simulink model "Longitudinal"  (R2025b)
settings: Solver=VariableStepAuto  StartTime=0.0  StopTime=5  MaxStep=0.001  RelTol=1e-3
undefined symbols (not defined in the file): car, rad, s, Tau_1, Tau_2, Tau_3, Tau_4, Tau_EM, tyre
libraries: aerolibconvert2 x3, simulink x2, autolibcoupling x1
(part 3 of 3)

== matlab function Longitudinal/longitudinal dynamics/Kinematics/Subsystem/Damper front/MATLAB Function ==
  data: x_dot input; x_dot_comp output; x_dot_reb output
function [ x_dot_comp , x_dot_reb ] = conv_x_dot(x_dot)

if x_dot > 0 
    x_dot_comp = x_dot; 
    x_dot_reb = 0;
else 
    x_dot_comp = 0;
    x_dot_reb = - x_dot;
end

== matlab function Longitudinal/longitudinal dynamics/Kinematics/Subsystem/Rear damping/MATLAB Function ==
  data: x_dot input; x_dot_comp output; x_dot_reb output
function [ x_dot_comp , x_dot_reb ] = conv_x_dot(x_dot)

if x_dot > 0 
    x_dot_comp = x_dot; 
    x_dot_reb = 0;
else 
    x_dot_comp = 0;
    x_dot_reb = - x_dot;
end

== matlab function Longitudinal/longitudinal dynamics/Fx equilibrium ==
  data: Drag output; Fz_FL output; a input; Fz_RR output; Fz_RL output; Fz_FR output; delta_Fz output; v input; Cx input; Cz input; delta_wb_front input; delta_wb_rear input; Jr_tot input; car input; M_inerzia output
function [Drag, Fz_FL, Fz_RR, Fz_RL, Fz_FR, delta_Fz, M_inerzia] = fx_equilibrium(a, v, Cx, Cz, delta_wb_front, delta_wb_rear, Jr_tot, car)

wb = car.wb0 + delta_wb_front + delta_wb_rear; %m

Downforce = 0.5 * car.rho * Cz * car.frontal_area * v ^ 2; % downforce N
Drag = 0.5 * car.rho * Cx * car.frontal_area * v ^ 2; % drag N
M_aero = Drag * (car.h_cp - car.h_cog) - Downforce * (car.lf - car.x_cp); %Nm

delta_Fz = Drag * car.h_cog / wb + M_aero / wb; %N
delta_Fz=delta_Fz/2;

M_inerzia = car.m * a * car.h_cog;
%J_f è di una singola ruota
%J_r totale da ruota a motore ICE
Fz_front = - Drag * car.h_cog / wb + (car.m * car.g + Downforce) * (car.lr + delta_wb_rear - car.delta) / wb - M_aero / wb - car.J_f*2* a / (car.R * wb); %N  (verificare J_f*4 oppure J_f*2!!!!!!!!!!!)

Fz_rear = Drag * car.h_cog / wb + (car.m * car.g + Downforce) * (car.lf + delta_wb_front + car.delta) / wb + M_aero / wb + Jr_tot * a / (car.R * wb); %N

if Fz_front <= 0
    Fz_rear = Fz_rear + Fz_front;
    Fz_front = 0;
elseif Fz_rear <0 
    Fz_front = Fz_front + Fz_rear;
    Fz_rear = 0;
end

Fz_FR = Fz_front / 2 ;
Fz_FL = Fz_FR ;

Fz_RL = Fz_rear / 2;
Fz_RR = Fz_RL ;

== matlab function Longitudinal/longitudinal dynamics/Fx powertrain calculation/FL ==
  data: Fx_EM_FL output; T input; T_b input; Fz input; a input; car input; delta_z_tyre_FL input
function Fx_EM_FL = fcn( T,T_b, Fz, a, car, delta_z_tyre_FL)

Fx_EM_FL = ( T - T_b - Fz * car.delta - car.J_f * a / ( car.R - delta_z_tyre_FL ) ) / ( car.R - delta_z_tyre_FL ) ; %N
% J - parameter for each tyre - J_f & J_r

== matlab function Longitudinal/Tyres/Rear Right ==
  data: tyre_RR input; Fx output; Fy output
function [Fx, Fy] = fcn(tyre_RR)

y = u;

== matlab function Longitudinal/Tyres/Front Right ==
  data: SR input; tyre input; Fx output; p input; Fz input; camber input
function Fx = fcn(SR,tyre,p,Fz,camber)

% PAC2002 puro longitudinale (Fx vs k)

     Fz0 = tyre.Fz0;
     if Fz0 == 0, Fz0 = max(1, Fz); end
    dfz = (Fz - Fz0)/Fz0;

    pi0 = tyre.pi0;  % Pa nominale
    dpi = (p - pi0)/pi0;
    
    Cx1 = tyre.Cx1;
    Dx1 = tyre.Dx1;
    Dx2 = tyre.Dx2;
    Dx3 = tyre.Dx3;
    Ex1 = tyre.Ex1;
    Ex2 = tyre.Ex2;
    Ex3 = tyre.Ex3;
    Ex4 = tyre.Ex4;
    Kx1 = tyre.Kx1;
    Kx2 = tyre.Kx2;
    Kx3 = tyre.Kx3;
    Hx1 = tyre.Hx1;
    Hx2 = tyre.Hx2;
    Vx1 = tyre.Vx1;
    Vx2 = tyre.Vx2;
    px1 = tyre.px1;
    px2 = tyre.px2;
    px3 = tyre.px3;
    px4 = tyre.px4;
    lmux = tyre.lmux;

    gamma = camber*pi/180;
    mu = (Dx1 + Dx2*dfz) * (1 - Dx3*(gamma^2)) * (1 + px3*dpi + px4*dpi^2)*lmux;
    % mu = 1.4;

    D = mu * Fz;
    C = Cx1;
    K = Fz * (Kx1 + Kx2*dfz) * exp(Kx3*dfz) * (1 + px1*dpi + px2*dpi^2);
    B = K / (C*D + eps);

    SH = Hx1 + Hx2*dfz;
    SR  = SR + SH;

    E  = (Ex1 + Ex2*dfz + Ex3*dfz^2) * (1 - Ex4*sign(SR));
    SV = Fz * (Vx1 + Vx2*dfz);

    Fx0 = D * sin( C * atan( B*SR - E*(B*SR - atan(B*SR)) ) );
    Fx = Fx0 + SV;

== matlab function Longitudinal/Tyres/Rear Left ==
  data: tyre_RL input; Fx output; Fy output
function [Fx, Fy] = fcn(tyre_RL)

y = u;

== matlab function Longitudinal/longitudinal dynamics/Kinematics/RL/Rear Left Tyre ==
  data: car input; wheel_travel_RL output; IR_RL input; AS_RL input; Fz_RL input; h_ground_RL output; delta_Fz input; delta_z_tyre_RL output; a input
function [wheel_travel_RL, h_ground_RL, delta_z_tyre_RL]      = kinematics(car, IR_RL, AS_RL, Fz_RL, delta_Fz, a)

delta_z_tyre_RL = Fz_RL / car.k_tyre/1000; % tyre vertical stiffness - kz_tyre - for front and rear tyres, look at buses
k_spring_ground_RL = (car.k_spring_rear * IR_RL^2);

if a > 0 % under acceleration
    delta_z_spring_RL = (Fz_RL - delta_Fz) / k_spring_ground_RL + delta_Fz * ((1-AS_RL/100)/k_spring_ground_RL) ; % rear axle
else % under braking
    delta_z_spring_RL = Fz_RL / k_spring_ground_RL; % rear axle
end

%wheel center movement only due to spring deflection at ground. 
%to be used in the kineamtics block (camber, antidive, ir,...)
wheel_travel_RL = delta_z_spring_RL - car.z0_spring_rear; % if negative it is bounce

%to be used to find the new height of the car from the ground
jounce_RL = delta_z_tyre_RL + delta_z_spring_RL - car.z0_rear;
h_ground_RL = car.h0_ground_rear - jounce_RL;
